simulink model "discrete_Hinf_control"  (R2017b)
settings: Solver=FixedStepDiscrete  StartTime=0.0  StopTime=15  FixedStep=Ts  RelTol=1e-3
values from neighbouring files (symbols this model uses):
  c_FIR = zeros(1,n)    [input_shaping.m]
  cd_den_clean = cell2mat(den_clean)    [controller_design.m]
  cd_num_clean = cell2mat(num_clean)    [controller_design.m]
  d_den = cell2mat(sysd.den)    [controller_design.m]
  d_num = cell2mat(sysd.num)    [controller_design.m]
  Ts = 1/fs    (= 0.001)    [demo.m]
settings Model: Creator=hasee  LastModifiedBy=hasee

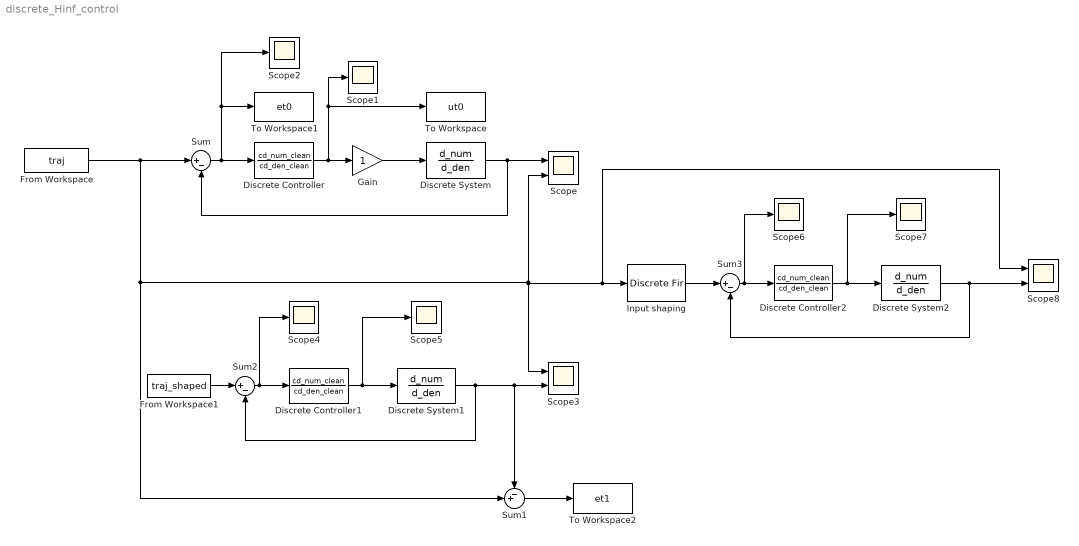
== system discrete_Hinf_control ==
  Discrete Controller : DiscreteTransferFcn  Numerator=cd_num_clean  Denominator=cd_den_clean  SampleTime=Ts
  Discrete Controller1 : DiscreteTransferFcn  Numerator=cd_num_clean  Denominator=cd_den_clean  SampleTime=Ts
  Discrete Controller2 : DiscreteTransferFcn  Numerator=cd_num_clean  Denominator=cd_den_clean  SampleTime=Ts
  Discrete System : DiscreteTransferFcn  Numerator=d_num  Denominator=d_den
  Discrete System1 : DiscreteTransferFcn  Numerator=d_num  Denominator=d_den
  Discrete System2 : DiscreteTransferFcn  Numerator=d_num  Denominator=d_den
  From Workspace : FromWorkspace  VariableName=traj  SampleTime=0.001
  From Workspace1 : FromWorkspace  VariableName=traj_shaped  SampleTime=0.001
  Gain : Gain
  Input shaping : DiscreteFir  Coefficients=c_FIR
  Scope : Scope  NumInputPorts=2
  Scope{1..2,4..7} (6 alike) : Scope
  Scope3 : Scope  NumInputPorts=2
  Scope8 : Scope  NumInputPorts=2
  Sum : Sum  Inputs=|+-
  Sum1 : Sum  Inputs=-+|
  Sum2 : Sum  Inputs=|+-
  Sum3 : Sum  Inputs=|+-
  To Workspace : ToWorkspace  VariableName=ut0  SaveFormat=Structure With Time  SampleTime=-1
  To Workspace1 : ToWorkspace  VariableName=et0  SaveFormat=Structure With Time  SampleTime=-1
  To Workspace2 : ToWorkspace  VariableName=et1  SaveFormat=Structure With Time  SampleTime=-1
  wires:
  Discrete Controller/1 -> To Workspace/1, Scope1/1, Gain/1
  Gain/1 -> Discrete System/1
  Sum/1 -> Scope2/1, To Workspace1/1, Discrete Controller/1
  Discrete System/1 -> Scope/1, Sum/2
  From Workspace/1 -> Sum1/2, Scope8/1, Input shaping/1, Scope3/1, Scope/2, Sum/1
  Sum1/1 -> To Workspace2/1
  Discrete System1/1 -> Sum2/2, Scope3/2, Sum1/1
  Discrete Controller1/1 -> Scope5/1, Discrete System1/1
  From Workspace1/1 -> Sum2/1
  Sum2/1 -> Scope4/1, Discrete Controller1/1
  Discrete System2/1 -> Scope8/2, Sum3/2
  Sum3/1 -> Scope6/1, Discrete Controller2/1
  Input shaping/1 -> Sum3/1
  Discrete Controller2/1 -> Scope7/1, Discrete System2/1
